simulink model "Lift_model"  (R2021a)
settings: Solver=VariableStepAuto  StartTime=0.0  StopTime=30  RelTol=1e-3
model workspace: external: MAT-File (data not in the file)
values from neighbouring files (symbols this model uses):
  Cur_Floor = 0    [Run_Simulink.m]
  Req_Floor = 5    [Run_Simulink.m]
settings Model: EnablePacing=on  OrderedModelArguments=off  Creator=bunce  LastModifiedBy=matteopenlington

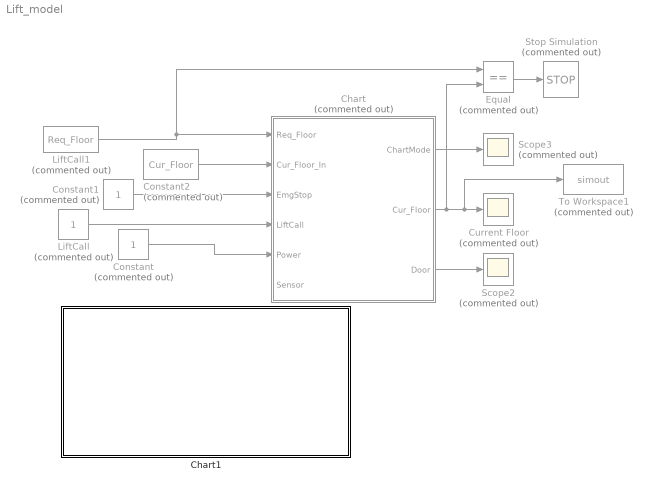
== system Lift_model ==
  Chart : Stateflow chart  Commented=on  TreatAsAtomicUnit=on
      settings: PortSchema="{\"entries\":[{\"content\":{\"sides\":[{\"content\":{\"connectorIds\":[\"In3\",\"In2\",\"In1\",\"In4\",\"In5\",\"In6\"]},\"type\":\"ConnectorPlacement.EquallySpacedRectSide\",\"uuid\":\"c8bed834-1690-4efd-86a4-97cdd0f25b0a\"},{\"content\":{\"connectorIds\":[\"Out1\",\"Out2\",\"Out3\"],\"side\":\"RIGHT\"},\"type\":\"ConnectorPlacement.EquallySpacedRectSide\",\"uuid\":\"9be9dadd-44ba-4f87-9487-5eee97fcd502\"},{\"content\":{\"connectorIds\":[],\"side\":\"TOP\"},\"type\":\"ConnectorPlacement.EquallySpacedRectSide\",\"uuid\":\"56706cb4-3cbd-4717-af64-550608b78a0a\"}]},\"type\":\"ConnectorPlacement.EquallySpacedConnector\",\"uuid\":\"4a7e4f94-8a4d-46c5-b98f-186c0a2fba81\"}],\"packageUris\":[\"http://schema.mathworks.com/mf0/Connector/R2020b\"],\"version\":\"1.0\"}"
  Chart1 : Stateflow chart  TreatAsAtomicUnit=on
  Constant : Constant  Commented=on
  Constant1 : Constant  Commented=on
  Constant2 : Constant  Commented=on  Value=Cur_Floor
  Current Floor : Scope  Commented=on
  Equal : RelationalOperator  Commented=on  Operator===  OutDataTypeStr=boolean  RndMeth=Simplest
  LiftCall : Constant  Commented=on
  LiftCall1 : Constant  Commented=on  Value=Req_Floor
  Scope2 : Scope  Commented=on
  Scope3 : Scope  Commented=on
  Stop Simulation : Stop  Commented=on
  To Workspace1 : ToWorkspace  Commented=on  VariableName=simout  SampleTime=-1
  wires:
  Constant/1 -> Chart/5(Power)
  LiftCall1/1 -> Equal/1, Chart/3(Req_Floor)
  LiftCall/1 -> Chart/4(LiftCall)
  Chart/2(Cur_Floor) -> Equal/2, To Workspace1/1, Current Floor/1
  Chart/1(ChartMode) -> Scope3/1
  Chart/3(Door) -> Scope2/1
  Constant1/1 -> Chart/1(EmgStop)
  Equal/1 -> Stop Simulation/1
  Constant2/1 -> Chart/2(Cur_Floor_In)

== stateflow chart Lift_model/Chart1 ==
  state InterfaceFromApp
    entry:
    coder.extrinsic('Copy_of_App_interface');
    app = Copy_of_App_interface(this);
    initialiseData();
    state initialiseData [function]
      (default) -> (junction 12) : {
          | CurFloor = 0;
          | RqFloor = 0;
          | }
  (default) -> InterfaceFromApp
  data: app local

== stateflow chart Lift_model/Chart ==
  state Initial
    entry:
    Cur_Floor = Cur_Floor_In
    %Cur_Floor = 0;
    %Sensor = 0;
  note: This is for:
      | - lift is at floor 0.
      | - user calls lift from floor 0
      | - lift requested to floor 2
  state Idle_doors
    entry:
    exit:
    state DoorOpen
      entry:
      Door = 1;
    state DoorClose
      entry:
      Door = 0;
    (default) -> DoorOpen
    DoorClose -> DoorOpen [order 1] : [Door == 0 || Sensor == 1]
    DoorOpen -> DoorClose : [Door == 1]
    DoorClose -> Idle_doors [order 2] : [Door == 0 && Sensor == 0]
  state Idle_waiting
  state MovingUp
    entry:
    %Motor == 1;
    exit:
    %Motor == 0;
  state MovingDown
    entry:
    %Motor == -1;
    exit:
    %Motor == 0;
  (default) -> Initial
  Initial -> (junction 55)
  (junction 55) -> Idle_waiting [order 2] : [LiftCall ~= 1]
  (junction 55) -> Idle_doors [order 1] : [LiftCall == 1]
  Idle_doors -> MovingUp [order 1] : [Req_Floor > Cur_Floor]
  MovingUp -> Idle_doors : after(2,sec){Cur_Floor = Cur_Floor + 1}
  Idle_doors -> MovingDown [order 2] : [Req_Floor < Cur_Floor]
  MovingDown -> Idle_doors : after(2,sec){Cur_Floor = Cur_Floor - 1}
  data: ChartMode output Enum: ChartModeType; Cur_Floor output; EmgStop input; Cur_Floor_In input; Req_Floor input; LiftCall input; Power input; Sensor input; Door output
